simulink model "BPSExampleFlightSim"  (R2017b)
settings: Solver=VariableStepAuto  StartTime=0.0  StopTime=14  RelTol=1e-3
settings Model: Creator=Joe  LastModifiedBy=Joe

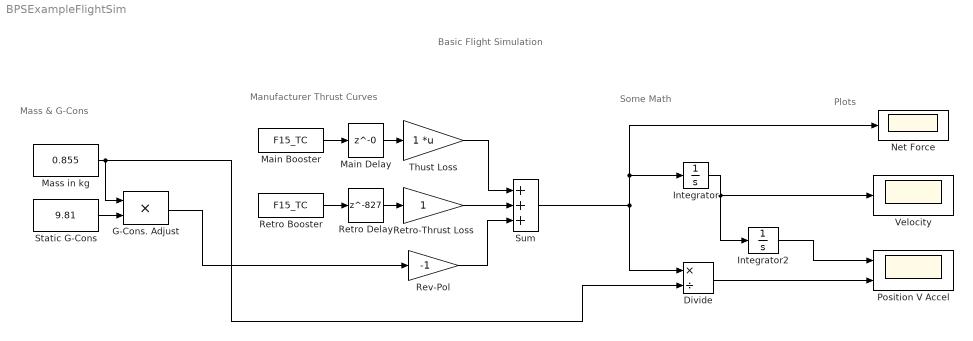
== system BPSExampleFlightSim ==
  note: Mass & G-Cons
  note: Manufacturer Thrust Curves
  note: Basic Flight Simulation
  note: Plots
  note: Some Math
  Divide : Product  Inputs=*/
  G-Cons. Adjust : Product  Inputs=**
  Integrator : Integrator
  Integrator2 : Integrator
  Main Booster : FromWorkspace  VariableName=F15_TC  OutputAfterFinalValue=Setting to zero
  Main Delay : Delay  DelayLength=0
  Mass in kg : Constant  Value=0.855
  Net Force : Scope
  Position V Accel : Scope  NumInputPorts=2
  Retro Booster : FromWorkspace  VariableName=F15_TC  OutputAfterFinalValue=Setting to zero
  Retro Delay : Delay  DelayLength=827  SampleTime=0.01
  Retro-Thrust Loss : Gain
  Rev-Pol : Gain  Gain=-1
  Static G-Cons : Constant  Value=9.81
  Sum : Sum  Inputs=+++
  Thust Loss : Gain  Multiplication=Matrix(K*u)
  Velocity : Scope
  wires:
  Thust Loss/1 -> Sum/1
  Divide/1 -> Position V Accel/2
  Mass in kg/1 -> G-Cons. Adjust/1, Divide/2
  Integrator/1 -> Velocity/1, Integrator2/1
  Static G-Cons/1 -> G-Cons. Adjust/2
  Rev-Pol/1 -> Sum/3
  Integrator2/1 -> Position V Accel/1
  Retro Delay/1 -> Retro-Thrust Loss/1
  Retro-Thrust Loss/1 -> Sum/2
  Main Booster/1 -> Main Delay/1
  G-Cons. Adjust/1 -> Rev-Pol/1
  Sum/1 -> Divide/1, Net Force/1, Integrator/1
  Main Delay/1 -> Thust Loss/1
  Retro Booster/1 -> Retro Delay/1
